simulink model "Prob2"  (R2022a)
settings: Solver=VariableStepAuto  StartTime=0.0  StopTime=5  RelTol=1e-3
values from neighbouring files (symbols this model uses):
  A = [-4 -2.5; 4 0]    [Examen_2_prob2.m]
  B = [1; 0]    [Examen_2_prob2.m]
  C = [1 0.75]    [Examen_2_prob2.m]
  K = Ks_LQR(1:2)    [Examen_2_prob2.m]
  Ki = -Ks_LQR(3)    [Examen_2_prob2.m]
settings Model: Creator=earaya  LastModifiedBy=ranvargas
settings DataIOCC: ReturnWorkspaceOutputs=off

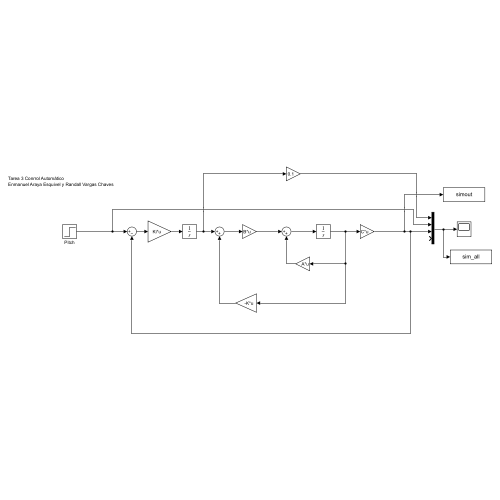
[thumbnail: Simulink's stored preview of the top-level diagram]
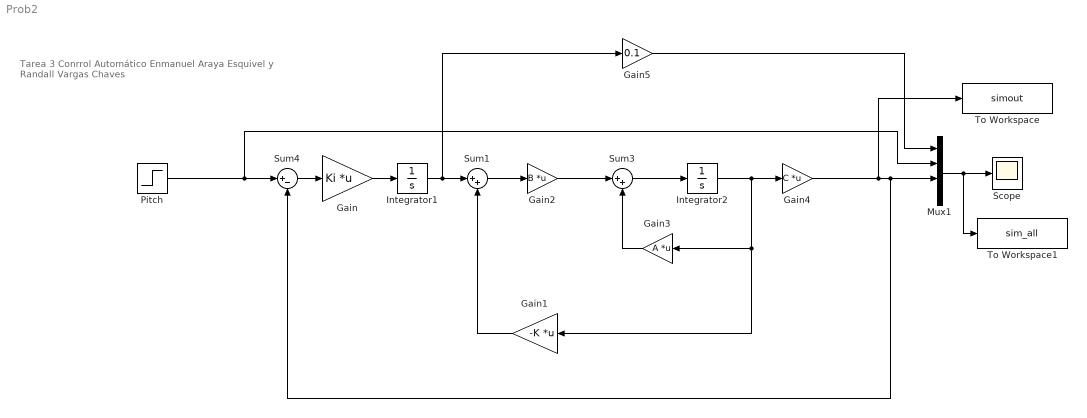
== system Prob2 ==
  note: Tarea 3 Conrrol Automático
      | Enmanuel Araya Esquivel y Randall Vargas Chaves
  Gain : Gain  Gain=Ki  Multiplication=Matrix(K*u)
  Gain1 : Gain  Gain=-K  Multiplication=Matrix(K*u)
  Gain2 : Gain  Gain=B  Multiplication=Matrix(K*u)
  Gain3 : Gain  Gain=A  Multiplication=Matrix(K*u)
  Gain4 : Gain  Gain=C  Multiplication=Matrix(K*u)
  Gain5 : Gain  Gain=0.1
  Integrator1 : Integrator
  Integrator2 : Integrator
  Mux1 : Mux
  Pitch : Step  Time=0  SampleTime=0
  Scope : Scope
  Sum1 : Sum  Inputs=|++
  Sum3 : Sum  Inputs=|++
  Sum4 : Sum  Inputs=|+-
  To Workspace : ToWorkspace  VariableName=simout  SaveFormat=Timeseries  SampleTime=-1
  To Workspace1 : ToWorkspace  VariableName=sim_all  SaveFormat=Timeseries  SampleTime=-1
  wires:
  Gain2/1 -> Sum3/1
  Mux1/1 -> To Workspace1/1, Scope/1
  Integrator2/1 -> Gain3/1, Gain1/1, Gain4/1
  Sum4/1 -> Gain/1
  Integrator1/1 -> Gain5/1, Sum1/1
  Gain3/1 -> Sum3/2
  Gain/1 -> Integrator1/1
  Gain1/1 -> Sum1/2
  Gain5/1 -> Mux1/1
  Sum1/1 -> Gain2/1
  Gain4/1 -> To Workspace/1, Mux1/3, Sum4/2
  Sum3/1 -> Integrator2/1
  Pitch/1 -> Mux1/2, Sum4/1
